simulink model "simu2_taller_2"  (R2023b)
settings: Solver=VariableStepAuto  StartTime=0.0  StopTime=10  RelTol=1e-3
settings Model: Creator=ASUS  LastModifiedBy=ASUS

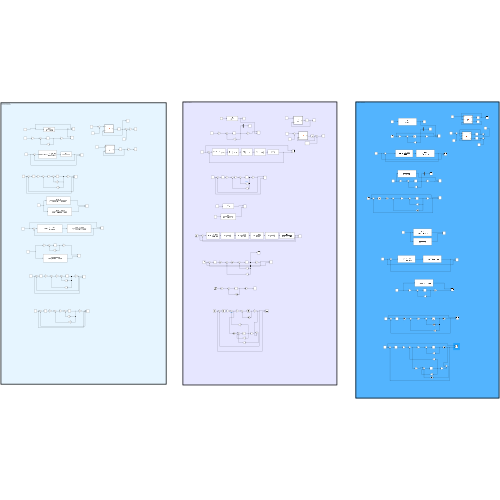
[thumbnail: Simulink's stored preview of the top-level diagram]
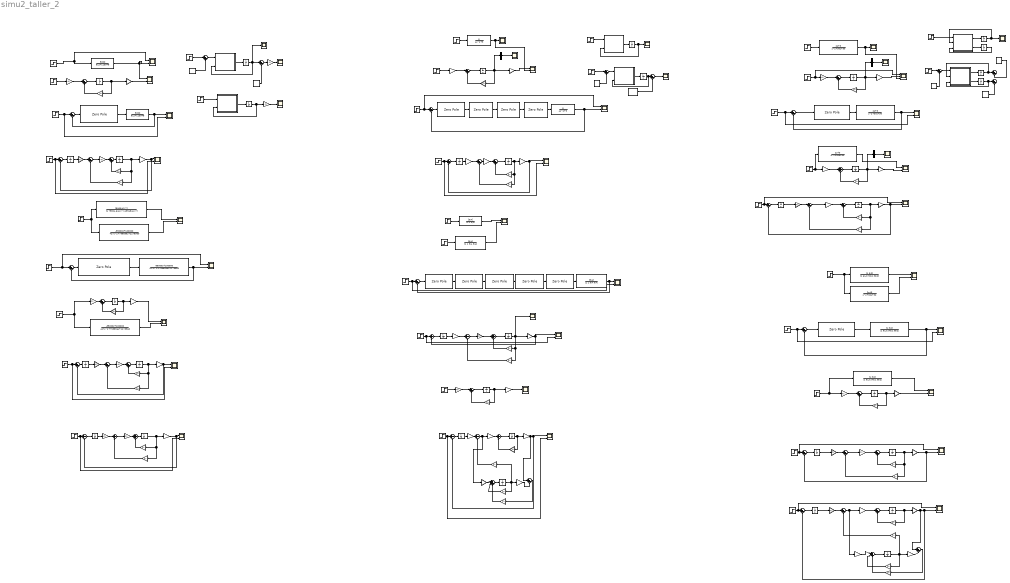
== system simu2_taller_2 ==
  note: CUARTO PUNTO
      | TALLER ORIGINAL
  note: PRIMER PUNTO
  note: CUARTO PUNTO
  Constant : Constant  Value=-1.578
  Constant1 : Constant  Value=12
  Constant2 : Constant  Value=1.5707
  Constant3 : Constant
  Constant4 : Constant  Value=7.84
  Constant5 : Constant
  Constant6 : Constant
  Gain{,5,57,69} (4 alike) : Gain  Gain=[5/4 ;0]  Multiplication=Matrix(K*u)
  Gain{1,4,18,21,42,44,56,63,68,73} (10 alike) : Gain  Gain=[0 1]  Multiplication=Matrix(K*u)
  Gain10 : Gain  Gain=[172/5 2123/5 6441/5]  Multiplication=Matrix(K*u)
  Gain11 : Gain  Gain=[2;1/2]  Multiplication=Matrix(K*u)
  Gain12 : Gain  Gain=[5/4 ;0;0]  Multiplication=Matrix(K*u)
  Gain{7,13,26,31} (4 alike) : Gain  Gain=[0 0 1]  Multiplication=Matrix(K*u)
  Gain14 : Gain  Gain=[0 0 -9/4;1 0 -9/4; 0 1 -1]  Multiplication=Matrix(K*u)
  Gain15 : Gain  Gain=[1 0]  Multiplication=Matrix(K*u)
  Gain16 : Gain  Gain=[-29 2;-1/2 -1]  Multiplication=Matrix(K*u)
  Gain{17,20,62,72} (4 alike) : Gain  Gain=[3;2]  Multiplication=Matrix(K*u)
  Gain{19,22,65,74} (4 alike) : Gain  Gain=[0 -30;1 -30]  Multiplication=Matrix(K*u)
  Gain{2..3,55,67} (4 alike) : Gain  Gain=[0 -9/4;1 0]  Multiplication=Matrix(K*u)
  Gain23 : Gain  Gain=[938/927 1738/309]  Multiplication=Matrix(K*u)
  Gain24 : Gain  Gain=7360/309
  Gain25 : Gain  Gain=[3/2;1;0]  Multiplication=Matrix(K*u)
  Gain27 : Gain  Gain=[0 0 -30/2;1 0 -90/2; 0 1 -61/2]  Multiplication=Matrix(K*u)
  Gain28 : Gain  Gain=[-9413/3306 12167/204 4051/136]  Multiplication=Matrix(K*u)
  Gain29 : Gain  Gain=3200/3
  Gain30 : Gain  Gain=[3/2;1;0]  Multiplication=Matrix(K*u)
  Gain32 : Gain  Gain=[0 0 -30/2;1 0 -90/2; 0 1 -61/2]  Multiplication=Matrix(K*u)
  Gain33 : Gain  Gain=[5000/61]  Multiplication=Matrix(K*u)
  Gain34 : Gain  Gain=[1]  Multiplication=Matrix(K*u)
  Gain35 : Gain  Gain=[-113948/61]  Multiplication=Matrix(K*u)
  Gain36 : Gain  Gain=[5000/61]  Multiplication=Matrix(K*u)
  Gain37 : Gain  Gain=[1]  Multiplication=Matrix(K*u)
  Gain38 : Gain  Gain=[-113948/61]  Multiplication=Matrix(K*u)
  Gain39 : Gain  Gain=681135.56
  Gain40 : Gain  Gain=[-4.55]  Multiplication=Matrix(K*u)
  Gain41 : Gain  Gain=[100000/427; -35000/427]  Multiplication=Matrix(K*u)
  Gain43 : Gain  Gain=[0 -2278960/427; 1 -798856/427]  Multiplication=Matrix(K*u)
  Gain45 : Gain  Gain=[0 -2278960/427; 1 -798856/427]  Multiplication=Matrix(K*u)
  Gain46 : Gain  Gain=[100000/427; -35000/427]  Multiplication=Matrix(K*u)
  Gain47 : Gain  Gain=1.676018
  Gain48 : Gain  Gain=[0.000286 22.3614]  Multiplication=Matrix(K*u)
  Gain49 : Gain  Gain=-1
  Gain50 : Gain  Gain=-1
  Gain51 : Gain  Gain=[5000/61]  Multiplication=Matrix(K*u)
  Gain52 : Gain  Gain=[1]  Multiplication=Matrix(K*u)
  Gain53 : Gain  Gain=[-113948/61]  Multiplication=Matrix(K*u)
  Gain54 : Gain  Gain=681135.56
  Gain58 : Gain  Gain=256
  Gain59 : Gain  Gain=[19.2 75]  Multiplication=Matrix(K*u)
  Gain6 : Gain  Gain=[5/4 ;0;0]  Multiplication=Matrix(K*u)
  Gain60 : Gain  Gain=256
  Gain61 : Gain  Gain=[-4.55]  Multiplication=Matrix(K*u)
  Gain64 : Gain  Gain=[19.2 75]  Multiplication=Matrix(K*u)
  Gain66 : Gain  Gain=[938/927 1738/309]  Multiplication=Matrix(K*u)
  Gain70 : Gain  Gain=[6391/4;40]  Multiplication=Matrix(K*u)
  Gain71 : Gain  Gain=7360/309
  Gain75 : Gain  Gain=[1570;10]  Multiplication=Matrix(K*u)
  Gain8 : Gain  Gain=[0 0 -9/4;1 0 -9/4; 0 1 -1]  Multiplication=Matrix(K*u)
  Gain9 : Gain  Gain=5120
  Integrator{,1..34} (35 alike) : Integrator
  MATLAB Function : MATLAB Function  TreatAsAtomicUnit=on
  MATLAB Function1 : MATLAB Function  TreatAsAtomicUnit=on
  MATLAB Function2 : MATLAB Function  TreatAsAtomicUnit=on
  MATLAB Function3 : MATLAB Function  TreatAsAtomicUnit=on
  MATLAB Function4 : MATLAB Function  TreatAsAtomicUnit=on
  MATLAB Function5 : MATLAB Function  TreatAsAtomicUnit=on
  Mux : Mux  Inputs=1
  Mux1 : Mux  Inputs=1
  Mux2 : Mux  Inputs=1
  Scope{,3,8..10,12,14,28..33} (13 alike) : Scope
  Scope{1..2,4..7,13,15..27,34..36,66} (24 alike) : Scope  NumInputPorts=2
  Scope11 : Scope  NumInputPorts=3
  Step{,2..4,8,17..24,26..30,32} (19 alike) : Step  Time=0  SampleTime=0
  Step{1,5..7,9..16,25,31,33,45} (16 alike) : Step  SampleTime=0
  Sum{,3,5..6,9,11..13,15..16,19..20,22..23,25,27..28,31..33,35..36,39..40,42,44..45,47,49,51} (30 alike) : Sum  Inputs=|+-
  Sum{1..2,4,7..8,10,14,17..18,21,24,26,29..30,34,37..38,41,50} (19 alike) : Sum  Inputs=|++
  Sum43 : Sum  Inputs=|+++
  Sum46 : Sum  Inputs=|+++
  Transfer Fcn : TransferFcn  Numerator=[5]  Denominator=[4 0 9]
  Transfer Fcn1 : TransferFcn  Numerator=[5]  Denominator=[4 0 9]
  Transfer Fcn10 : TransferFcn  Numerator=[1 3/2]  Denominator=[1 61/2 90/2 30/2]
  Transfer Fcn11 : TransferFcn  Numerator=[1 3/2]  Denominator=[1 61/2 90/2 30/2]
  Transfer Fcn12 : TransferFcn  Numerator=[5000]  Denominator=[61 113948]
  Transfer Fcn13 : TransferFcn  Numerator=[5000]  Denominator=[61 113948]
  Transfer Fcn14 : TransferFcn  Numerator=[5000/42.7]  Denominator=[1 79824.6/42.7 113948/42.7]
  Transfer Fcn15 : TransferFcn  Numerator=[-35000 100000]  Denominator=[427 798856 2278960]
  Transfer Fcn16 : TransferFcn  Numerator=[-35000 100000]  Denominator=[427 798856 2278960]
  Transfer Fcn17 : TransferFcn  Numerator=[-35000 100000]  Denominator=[427 798856 2278960]
  Transfer Fcn2 : TransferFcn  Numerator=[5/4]  Denominator=[1 0 9/4]
  Transfer Fcn3 : TransferFcn  Numerator=[5/4]  Denominator=[1 1 9/4 9/4]
  Transfer Fcn{4,6..7,9} (4 alike) : TransferFcn  Numerator=[2 3]  Denominator=[1 30 30]
  Transfer Fcn5 : TransferFcn  Numerator=[5/4]  Denominator=[1 1 9/4 9/4]
  Transfer Fcn8 : TransferFcn  Numerator=[1 3/2]  Denominator=[1 61/2 90/2 30/2]
  Zero-Pole : ZeroPole  Zeros=[-2.34 ]  Poles=[0 -6.67]  Gain=[385.926]
  Zero-Pole1 : ZeroPole  Zeros=[-2.34 ]  Poles=[-6.67]
  Zero-Pole{7..10} (4 alike) : ZeroPole  Zeros=[-2.04 ]  Poles=[-7.85]
  Zero-Pole11 : ZeroPole  Zeros="[-2.23 -2.23 -2.23 -2.23 -2.23 -2.23  ]"  Poles=[0 -6.54 -6.54 -6.54 -6.54 -6.54 -6.54]  Gain=[1866.73]
  Zero-Pole12 : ZeroPole  Zeros=[-2.91 -2.91]  Poles=[0 -4.26 -4.26]  Gain=[29.55]
  Zero-Pole2 : ZeroPole  Zeros=[-2.34 ]  Poles=[-6.67]
  Zero-Pole3 : ZeroPole  Zeros=[-2.34 ]  Poles=[-6.67]
  Zero-Pole4 : ZeroPole  Zeros=[-2.80 -2.80]  Poles=[0 -5.72 -5.72]  Gain=[861.57]
  Zero-Pole5 : ZeroPole  Zeros=[-7144.95 ]  Poles=[0 -7814.01]  Gain=[716751.2192]
  Zero-Pole6 : ZeroPole  Zeros=[-2.04 ]  Poles=[0 -7.85]  Gain=[5030]
  wires:
  Step/1 -> Transfer Fcn/1
  Transfer Fcn1/1 -> Sum/2, Scope1/2
  Zero-Pole/1 -> Zero-Pole1/1
  Zero-Pole1/1 -> Zero-Pole2/1
  Zero-Pole2/1 -> Zero-Pole3/1
  Zero-Pole3/1 -> Transfer Fcn1/1
  Sum/1 -> Zero-Pole/1
  Step1/1 -> Sum/1, Scope1/1
  Step2/1 -> Gain/1
  Sum1/1 -> Integrator/1
  Gain/1 -> Sum1/1
  Integrator/1 -> Gain2/1, Gain1/1, Mux/1
  Gain1/1 -> Scope2/1
  Gain2/1 -> Sum1/2
  Mux/1 -> Scope3/1
  Transfer Fcn/1 -> Scope/1, Scope2/2
  Sum51/1 -> Gain5/1
  Integrator32/1 -> Gain4/1, Gain3/1, Gain64/1
  Gain5/1 -> Sum50/1
  Sum49/1 -> Integrator31/1
  Sum50/1 -> Integrator32/1
  Gain4/1 -> Scope66/1, Sum49/2
  Gain64/1 -> Sum51/2
  Step45/1 -> Sum49/1, Scope66/2
  Gain3/1 -> Sum50/2
  Integrator31/1 -> Gain60/1
  Gain60/1 -> Sum51/1
  Transfer Fcn2/1 -> Scope4/1
  Step3/1 -> Transfer Fcn2/1
  Step4/1 -> Transfer Fcn3/1
  Transfer Fcn3/1 -> Scope4/2
  Zero-Pole9/1 -> Zero-Pole10/1
  Zero-Pole8/1 -> Zero-Pole9/1
  Zero-Pole7/1 -> Zero-Pole8/1
  Zero-Pole6/1 -> Zero-Pole7/1
  Sum3/1 -> Zero-Pole6/1
  Step6/1 -> Scope6/2, Sum3/1
  Transfer Fcn5/1 -> Sum3/2, Scope6/1
  Zero-Pole10/1 -> Transfer Fcn5/1
  Gain8/1 -> Sum4/2
  Gain7/1 -> Sum5/2, Scope7/1
  Integrator1/1 -> Gain10/1, Gain8/1, Scope8/1, Gain7/1
  Gain6/1 -> Sum4/1
  Sum4/1 -> Integrator1/1
  Integrator2/1 -> Gain9/1
  Sum6/1 -> Gain6/1
  Gain9/1 -> Sum6/1
  Gain10/1 -> Sum6/2
  Sum5/1 -> Integrator2/1
  Step8/1 -> Gain12/1
  Sum7/1 -> Integrator3/1
  Gain12/1 -> Sum7/1
  Integrator3/1 -> Gain14/1, Gain13/1
  Gain13/1 -> Scope9/1
  Gain14/1 -> Sum7/2
  Step7/1 -> Sum5/1, Scope7/2
  Transfer Fcn7/1 -> Scope11/3, Scope10/1
  Mux1/1 -> Scope12/1
  Gain16/1 -> Sum8/2
  Gain15/1 -> Scope11/2
  Integrator4/1 -> Mux1/1, Gain15/1, Gain16/1
  Gain11/1 -> Sum8/1
  Sum8/1 -> Integrator4/1
  Step9/1 -> Transfer Fcn7/1
  Step10/1 -> Gain11/1, Scope11/1
  Step11/1 -> Scope13/2, Sum9/1
  Sum9/1 -> Zero-Pole11/1
  Transfer Fcn6/1 -> Scope13/1, Sum9/2
  Zero-Pole11/1 -> Transfer Fcn6/1
  Step5/1 -> Gain17/1, Transfer Fcn4/1
  Sum2/1 -> Integrator5/1
  Gain17/1 -> Sum2/1
  Integrator5/1 -> Gain19/1, Gain18/1, Mux2/1
  Gain18/1 -> Scope5/2
  Gain19/1 -> Sum2/2
  Mux2/1 -> Scope14/1
  Transfer Fcn4/1 -> Scope5/1
  Gain22/1 -> Sum10/2
  Gain21/1 -> Sum12/2, Scope15/2
  Integrator6/1 -> Gain21/1, Gain23/1, Gain22/1
  Gain20/1 -> Sum10/1
  Sum10/1 -> Integrator6/1
  Gain23/1 -> Sum11/2
  Step12/1 -> Scope15/1, Sum12/1
  Sum11/1 -> Gain20/1
  Integrator7/1 -> Gain24/1
  Gain24/1 -> Sum11/1
  Sum12/1 -> Integrator7/1
  Transfer Fcn8/1 -> Scope16/1
  Step13/1 -> Transfer Fcn9/1, Transfer Fcn8/1
  Transfer Fcn9/1 -> Scope16/2
  Transfer Fcn10/1 -> Sum13/2, Scope17/1
  Zero-Pole4/1 -> Transfer Fcn10/1
  Sum13/1 -> Zero-Pole4/1
  Step14/1 -> Scope17/2, Sum13/1
  Sum16/1 -> Integrator9/1
  Gain29/1 -> Sum15/1
  Integrator9/1 -> Gain29/1
  Step15/1 -> Sum16/1, Scope18/1
  Gain28/1 -> Sum15/2
  Gain26/1 -> Scope18/2, Sum16/2
  Gain32/1 -> Sum17/2
  Integrator10/1 -> Gain31/1, Gain32/1
  Gain30/1 -> Sum17/1
  Sum17/1 -> Integrator10/1
  Gain31/1 -> Scope19/2
  Transfer Fcn11/1 -> Scope19/1
  Step16/1 -> Transfer Fcn11/1, Gain30/1
  Sum15/1 -> Gain25/1
  Sum14/1 -> Integrator8/1
  Gain25/1 -> Sum14/1
  Gain27/1 -> Sum14/2
  Integrator8/1 -> Gain28/1, Gain27/1, Gain26/1
  Transfer Fcn12/1 -> Scope20/2, Scope21/1
  Step17/1 -> Transfer Fcn12/1, Scope20/1
  Gain35/1 -> Sum18/2
  Integrator11/1 -> Gain34/1, Gain35/1
  Gain33/1 -> Sum18/1
  Sum18/1 -> Integrator11/1
  Step18/1 -> Gain33/1
  Gain34/1 -> Scope21/2
  Step19/1 -> Scope22/2, Sum19/1
  Sum19/1 -> Zero-Pole5/1
  Zero-Pole5/1 -> Transfer Fcn13/1
  Transfer Fcn13/1 -> Sum19/2, Scope22/1
  Gain39/1 -> Sum22/1
  Integrator12/1 -> Gain39/1
  Step20/1 -> Scope23/2, Sum20/1
  Gain40/1 -> Sum22/2
  Gain37/1 -> Scope23/1, Sum20/2
  Sum20/1 -> Integrator12/1
  Sum22/1 -> Gain36/1
  Sum21/1 -> Integrator13/1
  Gain36/1 -> Sum21/1
  Integrator13/1 -> Gain37/1, Gain40/1, Gain38/1
  Gain38/1 -> Sum21/2
  Step21/1 -> Transfer Fcn14/1, Transfer Fcn15/1
  Transfer Fcn14/1 -> Scope24/1
  Transfer Fcn15/1 -> Scope24/2
  Sum23/1 -> Zero-Pole12/1
  Zero-Pole12/1 -> Transfer Fcn16/1
  Step22/1 -> Sum23/1, Scope25/1
  Transfer Fcn16/1 -> Scope25/2, Sum23/2
  Gain43/1 -> Sum24/2
  Integrator14/1 -> Gain43/1, Gain42/1
  Gain41/1 -> Sum24/1
  Sum24/1 -> Integrator14/1
  Step23/1 -> Transfer Fcn17/1, Gain41/1
  Gain42/1 -> Scope26/1
  Transfer Fcn17/1 -> Scope26/2
  Gain45/1 -> Sum26/2
  Integrator16/1 -> Gain48/1, Gain45/1, Gain44/1
  Gain46/1 -> Sum26/1
  Sum26/1 -> Integrator16/1
  Sum27/1 -> Gain46/1
  Sum25/1 -> Integrator15/1
  Gain44/1 -> Scope27/1, Sum25/2
  Gain48/1 -> Sum27/2
  Step24/1 -> Scope27/2, Sum25/1
  Integrator15/1 -> Gain47/1
  Gain47/1 -> Sum27/1
  MATLAB Function/1(vcp) -> Integrator17/1
  Integrator17/1 -> Scope28/1, Sum28/1, MATLAB Function/2(vc)
  Constant/1 -> Sum28/2
  Sum29/1 -> MATLAB Function/1(vin)
  Constant1/1 -> Sum29/2
  Step25/1 -> Sum29/1
  MATLAB Function1/1(vcp) -> Integrator18/1
  Integrator18/1 -> MATLAB Function1/2(vc), Gain49/1
  Step26/1 -> MATLAB Function1/1(vin)
  Gain49/1 -> Scope29/1
  Sum28/1 -> Gain50/1
  Gain50/1 -> Scope30/1
  Step27/1 -> MATLAB Function2/1(f)
  MATLAB Function2/1(tpp) -> Integrator19/1
  Integrator19/1 -> Scope31/1, MATLAB Function2/2(tp)
  MATLAB Function3/1(tpp) -> Integrator20/1
  Integrator20/1 -> MATLAB Function3/2(tp), Sum31/1
  Constant2/1 -> Sum31/2
  Constant4/1 -> Sum30/2
  Sum30/1 -> MATLAB Function3/1(f)
  Step28/1 -> Sum30/1
  Sum31/1 -> Scope32/1
  Step29/1 -> MATLAB Function4/1(vin)
  MATLAB Function4/1(vcp) -> Integrator21/1
  MATLAB Function4/2(ilp) -> Integrator22/1
  Integrator22/1 -> MATLAB Function4/3(il)
  Integrator21/1 -> Scope33/1, MATLAB Function4/2(vc)
  Integrator23/1 -> Sum32/1, MATLAB Function5/2(vc)
  MATLAB Function5/2(ilp) -> Integrator24/1
  MATLAB Function5/1(vcp) -> Integrator23/1
  Integrator24/1 -> Sum33/1, MATLAB Function5/3(il)
  Step30/1 -> Sum34/1
  Sum34/1 -> MATLAB Function5/1(vin)
  Constant3/1 -> Sum34/2
  Constant5/1 -> Sum33/2
  Constant6/1 -> Sum32/2
  Gain58/1 -> Sum39/1
  Integrator26/1 -> Gain58/1
  Gain55/1 -> Sum38/2
  Step31/1 -> Scope34/2, Sum36/1
  Gain59/1 -> Sum39/2
  Gain56/1 -> Sum44/1, Sum36/2, Scope34/1
  Sum38/1 -> Integrator27/1
  Sum36/1 -> Integrator26/1
  Gain57/1 -> Sum38/1
  Integrator27/1 -> Gain55/1, Gain56/1
  Sum39/1 -> Gain57/1, Gain69/1
  Integrator30/1 -> Gain59/1, Gain67/1, Gain68/1
  Gain69/1 -> Sum43/1
  Sum43/1 -> Integrator30/1
  Gain67/1 -> Sum43/2
  Gain70/1 -> Sum43/3
  Gain68/1 -> Sum44/2
  Sum44/1 -> Gain70/1
  Gain53/1 -> Sum37/2
  Integrator28/1 -> Gain53/1, Gain61/1, Gain52/1
  Gain51/1 -> Sum37/1
  Sum37/1 -> Integrator28/1
  Sum40/1 -> Gain51/1
  Sum35/1 -> Integrator25/1
  Gain52/1 -> Sum35/2, Scope35/1
  Gain61/1 -> Sum40/2
  Step32/1 -> Sum35/1, Scope35/2
  Integrator25/1 -> Gain54/1
  Gain54/1 -> Sum40/1
  Sum45/1 -> Integrator33/1
  Gain71/1 -> Sum42/1
  Integrator33/1 -> Gain71/1
  Step33/1 -> Sum45/1, Scope36/1
  Gain66/1 -> Sum42/2
  Sum41/1 -> Integrator29/1
  Gain62/1 -> Sum41/1
  Integrator29/1 -> Gain65/1, Gain63/1
  Gain63/1 -> Sum47/1, Scope36/2, Sum45/2
  Gain65/1 -> Sum41/2
  Gain74/1 -> Sum46/2
  Integrator34/1 -> Gain74/1, Gain66/1, Gain73/1
  Gain72/1 -> Sum46/1
  Sum46/1 -> Integrator34/1
  Sum42/1 -> Gain72/1, Gain62/1
  Gain73/1 -> Sum47/2
  Sum47/1 -> Gain75/1
  Gain75/1 -> Sum46/3

== matlab function simu2_taller_2/MATLAB Function1 ==
  data: vin input; vcp output; vc input
function vcp  = fcn(vin,vc)
R3=1000;
R2=220;
R1=10;
k1=R3/(R2*R1+R3*R1);
c=1*10e-3;

vcp=-1/(4*c)*vc-(vin*k1)/c;

== matlab function simu2_taller_2/MATLAB Function ==
  data: vin input; vcp output; vc input
function vcp  = fcn(vin,vc)
R3=1000;
R2=220;
R1=10;
k1=R3/(R2*R1+R3*R1);
c=1*10e-3;

vcp=-1/(4*c)*vc-(vin*k1)/c;

== matlab function simu2_taller_2/MATLAB Function2 ==
  data: f input; tpp output; tp input
function tpp = fcn(f,tp)
m=0.8;
g=9.8;
l=1;
k=10;


tpp=f/(m*l^2)-g/l*sin(tp)+k/(2*m)*sin(tp)*cos(tp);

== matlab function simu2_taller_2/MATLAB Function3 ==
  data: f input; tpp output; tp input
function tpp = fcn(f,tp)
m=0.8;
g=9.8;
l=1;
k=10;


tpp=f/(m*l^2)-g/l*sin(tp)+k/(2*m)*sin(tp)*cos(tp);

== matlab function simu2_taller_2/MATLAB Function4 ==
  data: vin input; vcp output; vc input; il input; ilp output
function [vcp,ilp] = fcn(vin,vc,il)
c=1/2;
L=2;
R=2;
ilp=vin-vc/L-2/L*il;
vcp=-1/(8*c)*vc^3+il/c+vin/c-vc/c;

== matlab function simu2_taller_2/MATLAB Function5 ==
  data: vin input; vcp output; vc input; il input; ilp output
function [vcp,ilp] = fcn(vin,vc,il)
c=1/2;
L=2;
R=2;
ilp=vin-vc/L-2/L*il;
vcp=-1/(8*c)*vc^3+il/c+vin/c-vc/c;
